simulink model "dents_scie_generation"  (R2015a)
settings: Solver=ode3  StartTime=0.0  StopTime=10*Tsw  FixedStep=1e-7  RelTol=1e-3
values from neighbouring files (symbols this model uses):
  Tsw = Ts * 10    (= 2e-05)    [VOC_param.m]    (also in power_control_param.m = 0.0002)
settings Model: Creator=rblan  LastModifiedBy=rblan

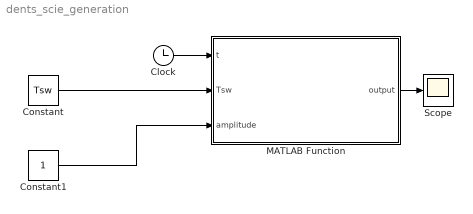
== system dents_scie_generation ==
  Clock : Clock
  Constant : Constant  Value=Tsw
  Constant1 : Constant
  MATLAB Function : MATLAB Function  TreatAsAtomicUnit=on
  Scope : Scope
  wires:
  Clock/1 -> MATLAB Function/1(t)
  Constant/1 -> MATLAB Function/2(Tsw)
  Constant1/1 -> MATLAB Function/3(amplitude)
  MATLAB Function/1(output) -> Scope/1

== matlab function dents_scie_generation/MATLAB Function ==
  data: t input; output output; Tsw input; amplitude input
function output = triangle(t,Tsw,amplitude)
%#codegen
%persistent signal ; 
persistent t_offset ; 

if isempty(t_offset) 
    t_offset = 0 ;  
end

if (t-t_offset>Tsw)
    t_offset = t ; 
    
end 

if ((t-t_offset)<=(Tsw/2))
    signal = -amplitude + (t-t_offset)*2*amplitude/(Tsw/2) ; 
   output = signal ;
   return 


else
    signal = 3*amplitude -  (t-t_offset)*2*amplitude/(Tsw/2) ; 
    output = signal ;
   return 
end 

end
